simulink model "SICARO"  (R2022b)
settings: Solver=ode23t  StartTime=0.0  StopTime=20  MaxStep=1e-3  RelTol=1e-3  AbsTol=1e-3
values from neighbouring files (symbols this model uses):
  air_rho = 1.225    [sicaro_inherited_params(stall).mat]
  battery_capacity = 22.8    [sicaro_inherited_params(stall).mat]
  CDO = 10.25    [sicaro_inherited_params(stall).mat]
  drag_linear = 0.002    [sicaro_inherited_params(stall).mat]
  drag_quad = 0.005    [sicaro_inherited_params(stall).mat]
  filtD_motor = 100    [sicaro_inherited_params(stall).mat]
  filtSpd_motor = 0.001    [sicaro_inherited_params(stall).mat]
  flap_radius = 0.05312    [sicaro_inherited_params(stall).mat]
  flap_surface_area = 0.025    [sicaro_inherited_params(stall).mat]
  kd_motor = 0    [sicaro_inherited_params(stall).mat]
  ki_motor = 0.00045    [sicaro_inherited_params(stall).mat]
  klinear = 0.03    [sicaro_inherited_params(stall).mat]
  kquad = 0.025    [sicaro_inherited_params(stall).mat]
  limit_motor = 0.25    [sicaro_inherited_params(stall).mat]
  monoco_mass = 160    [sicaro_inherited_params(stall).mat]
  monoco_prop =     [sicaro_inherited_params(stall).mat]
  monoco_radius = 0.61    [sicaro_inherited_params(stall).mat]
  monoco_wing =     [sicaro_inherited_params(stall).mat]
  monoco_wing_area = 0.239    [sicaro_inherited_params(stall).mat]
  waypoints = [-2 -2 0.14 -2 -2 6 0 0 6 2 0 6 ... (15 elements, 3x5)]    [sicaro_inherited_params(stall).mat]
undefined symbols (not defined in the file or in its folder): X, Y, Z
libraries: sm_lib x96, nesl_utility x38, slpidlib x20, fl_lib x12, sdl_lib x3, simulink x2, simulink_extras x1, batteryecm_lib x1, ee_lib x1
(part 7 of 7)

== matlab function SICARO/Collective Control/PD Alt Controller (Monoco positve direction clockwise)/Motor speed 2 thrust plot ==
  data: u input; y output
function y = fcn(u)
coder.extrinsic('fit');
input = u;

%disp (size(u));

%%%%% generate motor plot %%%%%%%%%%
% conversion2rads = 0.10471975513824;
% convert2Newton = 9.81/1000; 
% speed = conversion2rads.*[-31578 -31211 -30294 -29297 -28264 -27239 -26403 -25568 -24568 -23218 -21868 -20546 -19344 -18122 -16851 -15490 -13823 -11985 -8414 0 8414 11985 13823 15490 16851 18122 19334 20546 21868 23218 24568 25568 26403 27239 28264 29297 30294 31211 31578];
% speed = transpose(speed);
% thrust = convert2Newton.*[-485,-475,-450,-425,-400,-375,-350,-325,-300,-275,-250,-225,-200,-175,-150,-125,-100,-75,-50,0,50,75,100,125,150,175,200,225,250,275,300,325,350,375,400,425,450,475,485];
% thrust = transpose(thrust);
% f = fit(speed,thrust,'poly3'); % speed thrust function
% disp (f);
% disp (f(-10));
% plot(f,speed,thrust);
% xlabel('RPS')
% ylabel('Force')
% title('Motor plot force vs speed')

% rps = (100/2290).*[2290 2175.5 2061 1946.5 1832 1717.5 1603 1488.5 1374 1259.5 1145 1030.5 916];
% rps = transpose(rps);
% rot_freq = 0.1591549.*[30.2 28.82 27.5 26.21 24.95 23.71 22.5 21.3 20.13 18.97 17.82 16.67 15.5];
% rot_freq = transpose(rot_freq);
% g = fit(rps,rot_freq,'poly2');  % high thrust = high rotational freq = high lift
% disp(g);
% plot(g,rps,rot_freq);
% xlabel('thrust(%)')
% ylabel('rot_freq(hz)')
% title('thrust vs rot_freq')


x = input; 
func = 7.884e-11*x^3 - 7.663e-12*x^2 + 0.0006131*x + 8.695e-05; % motor speed(rps) vs thrust(N) ~ approximation, this value is the approx motor thrust obtained from motor rps 
y = func;


%y= 0;
% disp("func is");
% disp(y);
% disp("input is");
% disp(input);

== matlab function SICARO/Monowing/Speed Brake mode/Speed Brake Mode Activation ==
  data: rps input; y output; monoco_radius parameter; pitch input; air_rho parameter; monoco_wing_area parameter; Time input; Mode input
function y = fcn(rps, monoco_radius, pitch, air_rho, monoco_wing_area, Time, Mode)
linear_vel_sq = zeros(1,1);
linear_vel_sq = (rps * monoco_radius)^2;
drag_angle = 120;
drag_coeff = 0.1;



if Mode == 0
    if (pitch > drag_angle) && (Time < 8.0) 
        y = 0.5 * drag_coeff * air_rho * monoco_wing_area * linear_vel_sq * monoco_radius;
    else
        y = 0.0;
    end
else
    y = 0.0;
end

== matlab function SICARO/Monowing/Collective Control/Collective (Anhedral) ==
  data: Torque_negative input; Toggle input; output output
function output  = fcn(Torque_negative, Toggle)

if Toggle == 2.0
    output = Torque_negative * 1.0; % change this 
else
    output = 0.0;
end
%y = Torque_negative;

== matlab function SICARO/Monowing/Drag State/Drag filter ==
  data: drag input; Time input; drag_upper output; drag_lower output; Mode input
function [drag_upper, drag_lower] = fcn(drag, Time, Mode)
if Mode == 0
    if Time > 8.0 && Time < 12.0
        drag_upper = drag;
        drag_lower = 0.0;
    elseif Time > 12.0
        drag_lower = -1 * drag;
        drag_upper = 0.0;
    else
        drag_upper = drag;
        drag_lower = 0.0;
    end

elseif Mode == 1
    drag_upper = drag;
    drag_lower = 0.0;

else
    drag_upper = 0.0;
    drag_lower = -1 * drag;

end

== matlab function SICARO/Hover ==
  data: Y output; toggle_y output; X output; toggle_x output; Time input
function [Y, toggle_y, X, toggle_x] = fcn(Time)

sol_X = zeros(1,1);
sol_Toggle_Y = zeros(1,1);
sol_Toggle_X = zeros(1,1);
sol_Y = zeros(1,1);
Velocity = 0.2;

if Time > 10 && Time < 50
%     if Time > 10 && Time < 15
%         sol_X = 0;
%         sol_Toggle_Y = 1;
%         sol_Toggle_X = 1;
%         sol_Y = -1;
%     
%     elseif Time > 15 && Time < 20
%         sol_X = 0;
%         sol_Toggle_Y = 1;
%         sol_Toggle_X = 1;
%         sol_Y = 0;
%     
%     elseif Time > 20 && Time < 25
%         sol_X = 0;
%         sol_Toggle_Y = 1;
%         sol_Toggle_X = 1;
%         sol_Y = 1;
% 
%     elseif Time > 25 && Time < 30
%         sol_X = 0;
%         sol_Toggle_Y = 1;
%         sol_Toggle_X = 1;
%         sol_Y = 0;
%     end
% 
% else
    sol_X = 0;
    sol_Y = 0;
    sol_Toggle_Y = 1;
    sol_Toggle_X = 1;
end

Y = sol_Y;
X = sol_X;
toggle_y = sol_Toggle_Y;
toggle_x = sol_Toggle_X;

== matlab function SICARO/Monowing/Monowing_Assem/Old SICARO Controller For Translation/Collective & Cyclic Command Distribution (Disk Pitch) abt Yw ==
  data: u input; flap_dihedral_pitch_cmd output; gain_x input; heading input; Toggle input; Motor_Pulse output
function [flap_dihedral_pitch_cmd,Motor_Pulse] = fcn(u, gain_x, heading, Toggle)

if Toggle == 1 % Front Motor

    azimuth = u;
    %heading = deg2rad(heading);
    if ((abs(azimuth) - deg2rad(heading)) > pi/4) && ((abs(azimuth) - deg2rad(heading)) < 3*pi/4)
        tilt_xw = sin(azimuth - deg2rad(heading)); % tilt about yw heading in x direction 
        pitch = zeros(1,1);
        pitch = tilt_xw * gain_x; % only for cyclic y
        Motor_Pulse =  (pitch/abs(pitch)) * 1;

        if abs(pitch) > 0.60
            pitch = (pitch/abs(pitch)) * 0.60;
        end

        flap_dihedral_pitch_cmd = pitch;

    else
        
        Motor_Pulse =  0;
        flap_dihedral_pitch_cmd = 0.0;

    end

elseif Toggle == 2 % Back Motor

    azimuth = u;
    if (abs(azimuth) > pi/4) && (abs(azimuth) < 3*pi/4)
        tilt_xw = sin(azimuth + heading); % tilt around xw heading in y direction 
        pitch = zeros(1,1);
        pitch = tilt_xw * gain_x; % only for cyclic y
        Motor_Pulse =  (pitch/abs(pitch)) * 1;

        if abs(pitch) > 0.75
            pitch = (pitch/abs(pitch)) * 0.75;
        end

        flap_dihedral_pitch_cmd = pitch;

    else
        
        Motor_Pulse =  0;
        flap_dihedral_pitch_cmd = 0.0;

    end

else
    
    Motor_Pulse =  0;
    flap_dihedral_pitch_cmd = 0.0;

end





% kp = 1.3;
% desired_roll = 10;
% if (Annular_roll/abs(Annular_roll)) > 0.0
%     error_gain = kp*(Annular_roll - desired_roll);
% 
% elseif (Annular_roll/abs(Annular_roll)) < 0.0
%     error_gain = kp*(Annular_roll - (-1*desired_roll));
% 
% else
%     error_gain = 0.0;
% 
% end

% roll = gain * desired_flap * 2; % only for cyclic (original) 
% roll = desired_flap; % collective
% flap_cmd = roll - error_gain;

== matlab function SICARO/Monowing/Monowing_Assem/Old SICARO Controller For Translation/Cyclic Command Distribution ==
  data: pitch_gain_dihedral_front input; roll_gain_dihedral_front input; pitch_gain_dihedral_back input; roll_gain_dihedral_back input; Transition_Mode output; gain_x output; gain_y output; Dihedral_Mode output; Mode_Selection input
function [Transition_Mode, gain_x, gain_y, Dihedral_Mode] = fcn(pitch_gain_dihedral_front, roll_gain_dihedral_front, pitch_gain_dihedral_back, roll_gain_dihedral_back, Mode_Selection)

if Mode_Selection == 1
    Transition_Mode = 0;
    Dihedral_Mode = 1;
    gain_x = pitch_gain_dihedral_front;
    gain_y = roll_gain_dihedral_front;
else 
    Transition_Mode = 0;
    Dihedral_Mode = 2;
    gain_x = pitch_gain_dihedral_back;
    gain_y = roll_gain_dihedral_back;
end



% if Mode_Selection == 0
%     Transition_Mode = 1;
%     Dihedral_Mode = 0;
%     Anhedral_Mode = 0;
%     gain_x = 0;
%     gain_y = 0;
% elseif Mode_Selection == 1
%     Transition_Mode = 0;
%     Dihedral_Mode = 1;
%     Anhedral_Mode = 0;
%     gain_x = pitch_gain_dihedral;
%     gain_y = roll_gain_dihedral;
% elseif Mode_Selection == 2
%     Transition_Mode = 0;
%     Dihedral_Mode = 0;
%     Anhedral_Mode = 1;
%     gain_x = pitch_gain_anhedral;
%     gain_y = roll_gain_anhedral;
% else 
%     Transition_Mode = 0;
%     Dihedral_Mode = 0;
%     Anhedral_Mode = 0;
%     gain_x = 0;
%     gain_y = 0;
% end

== matlab function SICARO/Monowing/Collective Control/Collective Mode Switcher ==
  data: dihedral output; Time input; anhedral output; Mode input
function [dihedral,anhedral] = fcn(Time,Mode)
if Mode == 1
      dihedral = 1.0;
      anhedral = 0.0;
    
elseif Mode == 2
    dihedral = 1.0;
    anhedral = 0.0;
else
    dihedral = 0.0;
    anhedral = 0.0;
end


% if Mode == 0
%     
%     if Time > 8.0 && Time < 12.0
%         dihedral = 0.0; % upside cut torque
%         anhedral = 0.0;
%     elseif Time > 10
%         dihedral = 0.0;
%         anhedral = 1.0;
%     else
%         dihedral = 1.0;
%         anhedral = 0.0;
%     end
% 
% elseif Mode == 1
% 
%     dihedral = 1.0;
%     anhedral = 0.0;
% 
% elseif Mode == 2
% 
%     dihedral = 0.0;
%     anhedral = 1.0;
% 
% else
% 
%     dihedral = 0.0;
%     anhedral = 0.0;
% 
% end

== matlab function SICARO/Monowing/Horizontal Forces/Horizontal Motion X ==
  data: roll_in_deg input; force output; Lift input; flap_angle_data input; vx input; vy input; vz input; klinear parameter; kquad parameter; azimuth input; flap_angle input; desired_heading input; active_state output
function [force,active_state]  = fcn(roll_in_deg, Lift, flap_angle_data, vx, vy, vz, klinear, kquad, azimuth, flap_angle, desired_heading)
fx = zeros(1,1);
x = zeros(1,1);
v_l1 = zeros(1,1);
v_l2 = zeros(1,1);
roll_angle = abs(roll_in_deg);
%disp(Lift);
dihedral_offset = 2.0;
v_l1 = abs(vx) + abs(vy) + abs(vz);
v_l2 = sqrt(vx^2 + vy^2 + vz^2);

negative_x = 0;
positive_x = 1;
neutral_x = 2;
desired_heading = deg2rad(desired_heading);

if (azimuth - desired_heading) > 0 && flap_angle > 0 
    current_state = negative_x;
    active_state = 1;

elseif (azimuth - desired_heading) < 0 && flap_angle < 0
    current_state = negative_x;
    active_state = 2;
    
elseif (azimuth - desired_heading) > pi && flap_angle < 0
    current_state = negative_x;
    active_state = 3;

elseif (azimuth - desired_heading) > 0 && flap_angle < 0
    current_state = positive_x;
    active_state = 4;

elseif (azimuth - desired_heading) < 0 && flap_angle > 0
    current_state = positive_x;
    active_state = 5;

elseif (azimuth - desired_heading) > pi && flap_angle > 0
    current_state = positive_x;
    active_state = 6;

else
    current_state = neutral_x;
    active_state = 0;
end

%disp (current_state);
% disp (azimuth);
% disp (flap_angle);

% current_state = negative_y;

switch(current_state)

    case negative_x
        if roll_in_deg > 0 && roll_in_deg > dihedral_offset 
        %     if roll_in_deg > 0
            fx = Lift*sind(roll_in_deg-dihedral_offset);
            x = (-1*fx) + (kquad*v_l1*abs(vy) + klinear*abs(vy));
        elseif roll_in_deg < 0
            fx = Lift*sind(roll_angle);
            x = (-1*fx) + (kquad*v_l1*abs(vy) + klinear*abs(vy));
            %y = y  (kquad*v_l1*abs(vy) + klinear*abs(vy));
        else
            x = 0.0;
        end

    case positive_x
        if roll_in_deg > 0 && roll_in_deg > dihedral_offset 
        %     if roll_in_deg > 0
            fx = Lift*sind(roll_in_deg-dihedral_offset);
            x = fx - (kquad*v_l1*abs(vy) + klinear*abs(vy));
        elseif roll_in_deg < 0
            fx = Lift*sind(roll_angle);
            x = fx - (kquad*v_l1*abs(vy) + klinear*abs(vy));
            %y = y  (kquad*v_l1*abs(vy) + klinear*abs(vy));
        else
            x = 0.0;
        end

    case neutral_x 
            x = 0.0;

end

force = x;
% Acceleration_in_x_axis = x/monoco_mass;
% flap_angle_recording = flap_angle_data;

== matlab function SICARO/Monowing/Monowing_Assem/Old SICARO Controller For Translation/Collective & Cyclic Command Distribution (Disk Roll) abt Xw ==
  data: u input; flap_dihedral_roll_cmd output; gain_y input; heading input; Toggle input; Motor_Pulse output
function [flap_dihedral_roll_cmd,Motor_Pulse] = fcn(u, gain_y, heading, Toggle)

if Toggle == 1 % Front Motor

    azimuth = u;
    if (abs(azimuth) > 3*pi/4) || (abs(azimuth) < pi/4)
        tilt_yw = cos(azimuth + heading); % tilt around xw heading in y direction 
        roll = zeros(1,1);
        roll = tilt_yw * gain_y; % only for cyclic y
        Motor_Pulse =  (roll/abs(roll)) * 1;

        if abs(roll) > 0.6
            roll = (roll/abs(roll)) * 0.6;
        end

        flap_dihedral_roll_cmd = roll;

    else
        
        Motor_Pulse =  0;
        flap_dihedral_roll_cmd = 0.0;

    end

elseif Toggle == 2 % Back Motor

    azimuth = u;
    if (abs(azimuth) > 3*pi/4) || (abs(azimuth) < pi/4)
        tilt_yw = cos(azimuth + heading); % tilt around xw heading in y direction 
        roll = zeros(1,1);
        roll = tilt_yw * gain_y; % only for cyclic y
        Motor_Pulse =  (roll/abs(roll)) * 1;

        if abs(roll) > 0.6
            roll = (roll/abs(roll)) * 0.6;
        end

        flap_dihedral_roll_cmd = roll;

    else
        
        Motor_Pulse =  0;
        flap_dihedral_roll_cmd = 0.0;

    end

else
    
    Motor_Pulse =  0;
    flap_dihedral_roll_cmd = 0.0;

end







% kp = 1.3;
% desired_roll = 10;
% if (Annular_roll/abs(Annular_roll)) > 0.0
%     error_gain = kp*(Annular_roll - desired_roll);
% 
% elseif (Annular_roll/abs(Annular_roll)) < 0.0
%     error_gain = kp*(Annular_roll - (-1*desired_roll));
% 
% else
%     error_gain = 0.0;
% 
% end

% roll = gain * desired_flap * 2; % only for cyclic (original) 
% roll = desired_flap; % collective
% flap_cmd = roll - error_gain;

== matlab function SICARO/Cyclic Roll Control/PD Roll Controller (Monoco negative direction counter clockwise) Front Motor/Gain Switching ==
  data: aggro input; y output; Toggle input; annular_roll input; gentle input
function y = fcn(aggro, Toggle, annular_roll, gentle)

if Toggle > 0
    if abs(annular_roll) > 5.0
        y = aggro;
    else
        y = gentle;
    end
else
    y = 0;
end

% y = gentle;

== matlab function SICARO/Diamond ==
  data: Y output; toggle_y output; X output; toggle_x output; Time input; Z output
function [Y, toggle_y, X, toggle_x, Z] = fcn(Time)

sol_X = zeros(1,1);
sol_Toggle_Y = zeros(1,1);
sol_Toggle_X = zeros(1,1);
sol_Y = zeros(1,1);
Velocity = 0.35;

z = 2.3; 
if Time > 10 && Time < 37
    if Time > 10 && Time < 16
        sol_X = -2;
        sol_Toggle_Y = 1;
        sol_Toggle_X = 1;
        sol_Y = 2;
        z = 2.3; 
    
    elseif Time > 16 && Time < 27
        sol_X = 2;
        sol_Toggle_Y = 1;
        sol_Toggle_X = 1;
        sol_Y = 2;
        z = 2.0; 
    
    elseif Time > 27 && Time < 33
        sol_X = 0;
        sol_Toggle_Y = 1;
        sol_Toggle_X = 1;
        sol_Y = 0;
        z = 2.0; 
    end

else
    sol_X = 0;
    sol_Y = 0;
    sol_Toggle_Y = 0;
    sol_Toggle_X = 0;
end

Y = sol_Y;
X = sol_X;
Z = z;
toggle_y = sol_Toggle_Y;
toggle_x = sol_Toggle_X;

== matlab function SICARO/Motor speed 2 motor induced torque plot (Back Motor) ==
  data: u input; y output; Mode input
function y = fcn(u, Mode)
coder.extrinsic('fit');
input = u;

%disp (size(u));

%%%%% generate motor torque %%%%%%%%%%
% speed = [-8414 -11985 -13823 -15490 -16851 -18122 -19334 -20546 -21868 -23218 -24568 -25568 -26403 -27239 -28264 -29297 -30294 -31211 -31578 0 8414 11985 13823 15490 16851 18122 19334 20546 21868 23218 24568 25568 26403 27239 28264 29297 30294 31211 31578];
% %speed = transpose(speed);
% power = [-14.88 -21.18 -31 -41.67 -53.85 -66.98 -80.75 -94.53 -110.53 -127.1 -143.66 -161.84 -180.78 -199.72 -213.16 -226.38 -243.4 -268.51 -279.30 0 14.88 21.18 31 41.67 53.85 66.98 80.75 94.53 110.53 127.1 143.66 161.84 180.78 199.72 213.16 226.38 243.4 268.51 279.30];
% %power = transpose(power);
% torque = mrdivide(power,speed);
% %torque = transpose(torque);
% disp(torque);

% f = fit(speed,torque,'poly3'); % speed torque function
% disp (f);
% disp (f(-10));
% plot(f,speed,torque);
% xlabel('RPM')
% ylabel('Torque')
% title('Motor plot torque vs speed')


% conversion2rpm = 0.10471975513824;
% x = abs(input)/conversion2rpm; 
if Mode == 2
    y = 0.0031 * -1;  % dun change!
else
    y = 0.0031 * 0;
end
 
    
% y = 0.0066 * 0;

%y= 0;
% disp("func is");
% disp(y);
% disp("input is");
% disp(input);

== matlab function SICARO/Square Trajectory ==
  data: Y output; toggle_y output; X output; toggle_x output; Time input
function [Y, toggle_y, X, toggle_x] = fcn(Time)

sol_X = zeros(1,1);
sol_Toggle_Y = zeros(1,1);
sol_Toggle_X = zeros(1,1);
sol_Y = zeros(1,1);
Velocity = 0.2;

if Time > 6 && Time < 120
    if Time > 6 && Time < 16
        sol_X = 2;
        sol_Toggle_Y = 1;
        sol_Toggle_X = 1;
        sol_Y = 0;
    
    elseif Time > 16 && Time < 26
        sol_X = 2;
        sol_Toggle_Y = 1;
        sol_Toggle_X = 1;
        sol_Y = 4;
    
    elseif Time > 26 && Time < 36
        sol_X = -2;
        sol_Toggle_Y = 1;
        sol_Toggle_X = 1;
        sol_Y = 4;
    
    elseif Time > 32 && Time < 42
        sol_X = -2;
        sol_Toggle_Y = 1;
        sol_Toggle_X = 1;
        sol_Y = 0;
    
    elseif Time > 42 && Time < 50
        sol_X = 0;
        sol_Toggle_Y = 1;
        sol_Toggle_X = 1;
        sol_Y = 0;
    end

else
    sol_X = 0;
    sol_Y = 0;
    sol_Toggle_Y = 0;
    sol_Toggle_X = 0;
end

Y = sol_Y;
X = sol_X;
toggle_y = sol_Toggle_Y;
toggle_x = sol_Toggle_X;

== matlab function SICARO/Monowing/flap_moment  ==
  data: flap_angle input; y output; rps input; monoco_radius parameter; air_rho parameter; flap_surface_area parameter; flap_radius parameter
function y = fcn(flap_angle, rps, monoco_radius, air_rho, flap_surface_area, flap_radius)
linear_vel_sq = zeros(1,1);
linear_vel_sq = (rps * monoco_radius)^2;
y = flap_radius * 0.5 * 0.005 * flap_angle * air_rho * flap_surface_area * linear_vel_sq;

== matlab function SICARO/Motor speed 2 motor induced torque plot (Front Motor) ==
  data: u input; y output; Mode input
function y = fcn(u, Mode)
coder.extrinsic('fit');
input = u;

%disp (size(u));

%%%%% generate motor plot %%%%%%%%%%
% speed = [-8414 -11985 -13823 -15490 -16851 -18122 -19334 -20546 -21868 -23218 -24568 -25568 -26403 -27239 -28264 -29297 -30294 -31211 -31578 0 8414 11985 13823 15490 16851 18122 19334 20546 21868 23218 24568 25568 26403 27239 28264 29297 30294 31211 31578];
% %speed = transpose(speed);
% power = [-14.88 -21.18 -31 -41.67 -53.85 -66.98 -80.75 -94.53 -110.53 -127.1 -143.66 -161.84 -180.78 -199.72 -213.16 -226.38 -243.4 -268.51 -279.30 0 14.88 21.18 31 41.67 53.85 66.98 80.75 94.53 110.53 127.1 143.66 161.84 180.78 199.72 213.16 226.38 243.4 268.51 279.30];
% %power = transpose(power);
% torque = mrdivide(power,speed);
% %torque = transpose(torque);
% disp(torque);

% f = fit(speed,torque,'poly3'); % speed torque function
% disp (f);
% disp (f(-10));
% plot(f,speed,torque);
% xlabel('RPM')
% ylabel('Torque')
% title('Motor plot torque vs speed')


% conversion2rpm = 0.10471975513824;
% x = abs(input)/conversion2rpm; 
if Mode == 1
    y = 0.0031 * 1; % dun change!
else
    %y = 0.0066 * 0;
    y = 0.0031 * 0; 
end    
% y = 0.0066 * 0;

%y= 0;
% disp("func is");
% disp(y);
% disp("input is");
% disp(input);

== matlab function SICARO/Cyclic Roll Control/PD Pitch Controller (Monoco negative direction counter clockwise) Front Motor/Gain Switching2 ==
  data: aggro input; y output; Toggle input; annular_roll input; gentle input
function y = fcn(aggro, Toggle, annular_roll, gentle)

if Toggle > 0
    if abs(annular_roll) > 5.0
        y = aggro;
    else
        y = gentle;
    end
else
    y = 0;
end


% y = gentle;

== matlab function SICARO/Collective Control/PD Alt Controller (Monoco negative direction counter clockwise)/Motor Pulsing Filter ==
  data: u input; y output; toggle input
function y = fcn(u, toggle)

motor_pulse = zeros(1,1);

if toggle == 1
    motor_pulse = -1 * abs(u);
elseif toggle == -1
    motor_pulse = abs(u);
else
    motor_pulse = 0;
end

if abs(motor_pulse) > 300
    motor_pulse = motor_pulse/abs(motor_pulse) * 300;

end

y = motor_pulse;

== matlab function SICARO/Y Test ==
  data: Y output; toggle_y output; X output; toggle_x output; Time input
function [Y, toggle_y, X, toggle_x] = fcn(Time)

sol_X = zeros(1,1);
sol_Toggle_Y = zeros(1,1);
sol_Toggle_X = zeros(1,1);
sol_Y = zeros(1,1);
Velocity = 0.2;

if Time > 10 && Time < 40
   if Time > 10 && Time < 18
        sol_X = 0;
        sol_Toggle_Y = 1;
        sol_Toggle_X = 0;
        sol_Y = -2;
    
    elseif Time > 18 && Time < 30
        sol_X = 0;
        sol_Toggle_Y = 1;
        sol_Toggle_X = 0;
        sol_Y = 2;
    
    elseif Time > 30 && Time < 40
        sol_X = 0;
        sol_Toggle_Y = 1;
        sol_Toggle_X = 0;
        sol_Y = 0;
    end

else
    sol_X = 0;
    sol_Y = 0;
    sol_Toggle_Y = 1;
    sol_Toggle_X = 1;
end

Y = sol_Y;
X = sol_X;
toggle_y = sol_Toggle_Y;
toggle_x = sol_Toggle_X;

== matlab function SICARO/X Test ==
  data: Y output; toggle_y output; X output; toggle_x output; Time input
function [Y, toggle_y, X, toggle_x] = fcn(Time)

sol_X = zeros(1,1);
sol_Toggle_Y = zeros(1,1);
sol_Toggle_X = zeros(1,1);
sol_Y = zeros(1,1);
Velocity = 0.2;

if Time > 10 && Time < 40
    if Time > 10 && Time < 18
        sol_X = -2;
        sol_Toggle_Y = 0;
        sol_Toggle_X = 1;
        sol_Y = 0;
    
    elseif Time > 18 && Time < 30
        sol_X = 2;
        sol_Toggle_Y = 0;
        sol_Toggle_X = 1;
        sol_Y = 0;
    
    elseif Time > 30 && Time < 40
        sol_X = 0;
        sol_Toggle_Y = 0;
        sol_Toggle_X = 1;
        sol_Y = 0;
    end

else
    sol_X = 0;
    sol_Y = 0;
    sol_Toggle_Y = 0;
    sol_Toggle_X = 0;
end

Y = sol_Y;
X = sol_X;
toggle_y = sol_Toggle_Y;
toggle_x = sol_Toggle_X;

== matlab function SICARO/Cyclic Roll Control/PD Roll Controller (Monoco negative direction counter clockwise) Back Motor/Gain Switching ==
  data: aggro input; y output; Toggle input; annular_roll input; gentle input
function y = fcn(aggro, Toggle, annular_roll, gentle)

if Toggle > 0
    if abs(annular_roll) > 5
        y = aggro;
    else
        y = gentle;
    end
else
    y = 0;
end

% y = gentle;

== matlab function SICARO/Collective Control/PD Alt Controller (Monoco negative direction counter clockwise)/Motor speed 2 thrust plot ==
  data: u input; y output
function y = fcn(u)
coder.extrinsic('fit');
input = u;

%disp (size(u));

%%%%% generate motor plot %%%%%%%%%%
% conversion2rads = 0.10471975513824;
% convert2Newton = 9.81/1000; 
% speed = conversion2rads.*[-31578 -31211 -30294 -29297 -28264 -27239 -26403 -25568 -24568 -23218 -21868 -20546 -19344 -18122 -16851 -15490 -13823 -11985 -8414 0 8414 11985 13823 15490 16851 18122 19334 20546 21868 23218 24568 25568 26403 27239 28264 29297 30294 31211 31578];
% speed = transpose(speed);
% thrust = convert2Newton.*[-485,-475,-450,-425,-400,-375,-350,-325,-300,-275,-250,-225,-200,-175,-150,-125,-100,-75,-50,0,50,75,100,125,150,175,200,225,250,275,300,325,350,375,400,425,450,475,485];
% thrust = transpose(thrust);
% f = fit(speed,thrust,'poly3'); % speed thrust function
% disp (f);
% disp (f(-10));
% plot(f,speed,thrust);
% xlabel('RPS')
% ylabel('Force')
% title('Motor plot force vs speed')

% rps = (100/2290).*[2290 2175.5 2061 1946.5 1832 1717.5 1603 1488.5 1374 1259.5 1145 1030.5 916];
% rps = transpose(rps);
% rot_freq = 0.1591549.*[30.2 28.82 27.5 26.21 24.95 23.71 22.5 21.3 20.13 18.97 17.82 16.67 15.5];
% rot_freq = transpose(rot_freq);
% g = fit(rps,rot_freq,'poly2');  % high thrust = high rotational freq = high lift
% disp(g);
% plot(g,rps,rot_freq);
% xlabel('thrust(%)')
% ylabel('rot_freq(hz)')
% title('thrust vs rot_freq')


x = input; 
% prev % func = 7.884e-11*x^3 - 7.663e-12*x^2 + 0.0006131*x + 8.695e-05; % motor speed(rps) vs thrust(N) ~ approximation, this value is the approx motor thrust obtained from motor rps
func = 4.975e-11*x^3 + 3.747e-23*x^2 + 0.0003889*x - 3.142e-16;
y = func;


%y= 0;
% disp("func is");
% disp(y);
% disp("input is");
% disp(input);

== matlab function SICARO/Cyclic Roll Control/PD Pitch Controller (Monoco negative direction counter clockwise)2/Gain Switching2 ==
  data: aggro input; y output; Toggle input; annular_roll input; gentle input
function y = fcn(aggro, Toggle, annular_roll, gentle)

if Toggle > 0
    if abs(annular_roll) < 2.75
        y = aggro;
    else
        y = gentle;
    end
else
    y = 0;
end

== matlab function SICARO/Cyclic Roll Control/PD Pitch Controller (Monoco negative direction counter clockwise) Back Motor/Gain Switching2 ==
  data: aggro input; y output; Toggle input; annular_roll input; gentle input
function y = fcn(aggro, Toggle, annular_roll, gentle)

if Toggle > 0
    if abs(annular_roll) > 5.0
        y = aggro;
    else
        y = gentle;
    end
else
    y = 0;
end

% y = gentle;

== matlab function SICARO/Square Trajectory1 ==
  data: Y output; toggle_y output; X output; toggle_x output; Time input
function [Y, toggle_y, X, toggle_x] = fcn(Time)

sol_X = zeros(1,1);
sol_Toggle_Y = zeros(1,1);
sol_Toggle_X = zeros(1,1);
sol_Y = zeros(1,1);
Velocity = 0.2;

if Time > 6 && Time < 120
    if Time > 6 && Time < 16
        sol_X = 2;
        sol_Toggle_Y = 1;
        sol_Toggle_X = 1;
        sol_Y = 0;
    
    elseif Time > 16 && Time < 26
        sol_X = 2;
        sol_Toggle_Y = 1;
        sol_Toggle_X = 1;
        sol_Y = 4;
    
    elseif Time > 26 && Time < 36
        sol_X = -2;
        sol_Toggle_Y = 1;
        sol_Toggle_X = 1;
        sol_Y = 4;
    
    elseif Time > 32 && Time < 42
        sol_X = -2;
        sol_Toggle_Y = 1;
        sol_Toggle_X = 1;
        sol_Y = 0;
    
    elseif Time > 42 && Time < 50
        sol_X = 0;
        sol_Toggle_Y = 1;
        sol_Toggle_X = 1;
        sol_Y = 0;
    end

else
    sol_X = 0;
    sol_Y = 0;
    sol_Toggle_Y = 0;
    sol_Toggle_X = 0;
end

Y = sol_Y;
X = sol_X;
toggle_y = sol_Toggle_Y;
toggle_x = sol_Toggle_X;

== matlab function SICARO/Polar Test Front Motor ==
  data: mag_setpt output; Time input; desired_heading output; toggle output
function [mag_setpt, desired_heading, toggle] = fcn(Time)

mag = zeros(1,1);
heading = zeros(1,1);
cyclic_toggle = zeros(1,1);
% this is an exceptional example  

if Time > 10 && Time < 40
    cyclic_toggle = 1;
    if Time > 10 && Time < 18
        X_setpoint = -2;
        Y_setpoint = -2;
        mag = sqrt(X_setpoint^2 + Y_setpoint^2);
        
        % originally, supposed to be y as adjacent (due to matlab atan2
        % function structure), but this arrangement of
        % y being the opposite instead due to the swapping solves this issue 
        % atan2(x,y) swap to atan2(y,x)
        heading = atan2(Y_setpoint,X_setpoint);   

    elseif Time > 18 && Time < 26
        X_setpoint = 0-(-2);
        Y_setpoint = 0-(-2);
        mag = sqrt(X_setpoint^2 + Y_setpoint^2);

        % originally, supposed to be y as adjacent (due to matlab atan2
        % function structure), but this arrangement of
        % y being the opposite instead due to the swapping solves this issue 
        % atan2(x,y) swap to atan2(y,x)
        heading = atan2(Y_setpoint,X_setpoint);   
    
%     elseif Time > 26 && Time < 34
%         X_setpoint = 2;
%         Y_setpoint = -2;
%         mag = sqrt(X_setpoint^2 + Y_setpoint^2);
% 
%         % originally, supposed to be y as adjacent (due to matlab atan2
%         % function structure), but this arrangement of
%         % y being the opposite instead due to the swapping solves this issue 
%         % atan2(x,y) swap to atan2(y,x)
%         heading = atan2(Y_setpoint,X_setpoint);
% 
%      elseif Time > 34 && Time < 42
%         X_setpoint = -2;
%         Y_setpoint = 2;
%         mag = sqrt(X_setpoint^2 + Y_setpoint^2);
% 
%         % originally, supposed to be y as adjacent (due to matlab atan2
%         % function structure), but this arrangement of
%         % y being the opposite instead due to the swapping solves this issue 
%         % atan2(x,y) swap to atan2(y,x)
%         heading = atan2(Y_setpoint,X_setpoint);

    end
else
    cyclic_toggle = 0;
    mag = 0;
    heading = 0;
end
toggle = cyclic_toggle;
mag_setpt = mag;
desired_heading = heading;

== matlab function SICARO/Cyclic Roll Control/PD Control (Disk-Pitch Body-Roll Front Motor)/Gain Switching ==
  data: aggro input; y output; annular_roll input; gentle input; Toggle input
function y = fcn(aggro, annular_roll, gentle,Toggle)

if Toggle > 0
    if abs(annular_roll) > 5
        y = aggro;
    else
        y = gentle;
    end
else
    y = 0;
end

% y = gentle;

== matlab function SICARO/Cyclic Roll Control/Cartesian to polar transformation ==
  data: polar_feedback output; Y_fb input; X_fb input
function polar_feedback  = fcn(Y_fb,X_fb)

polarfb = zeros(1,1);
polarfb = sqrt(Y_fb^2 + X_fb^2);
polar_feedback = polarfb;

== matlab function SICARO/Monowing/Monowing_Assem/Disk-Pitch Body-Roll Command Distribution ==
  data: Disk_Pitch_Body_Roll_Front input; Disk_Pitch_Body_Roll_Back input; Transition_Mode output; gain output; Mode_Select output; Mode_Selection input
function [Transition_Mode, gain, Mode_Select] = fcn(Disk_Pitch_Body_Roll_Front,Disk_Pitch_Body_Roll_Back,Mode_Selection)

if Mode_Selection == 1
    Transition_Mode = 0;
    Mode_Select = 1;
    gain = Disk_Pitch_Body_Roll_Front;
else 
    Transition_Mode = 0;
    Mode_Select = 2;
    gain = Disk_Pitch_Body_Roll_Back;
end



% if Mode_Selection == 0
%     Transition_Mode = 1;
%     Dihedral_Mode = 0;
%     Anhedral_Mode = 0;
%     gain_x = 0;
%     gain_y = 0;
% elseif Mode_Selection == 1
%     Transition_Mode = 0;
%     Dihedral_Mode = 1;
%     Anhedral_Mode = 0;
%     gain_x = pitch_gain_dihedral;
%     gain_y = roll_gain_dihedral;
% elseif Mode_Selection == 2
%     Transition_Mode = 0;
%     Dihedral_Mode = 0;
%     Anhedral_Mode = 1;
%     gain_x = pitch_gain_anhedral;
%     gain_y = roll_gain_anhedral;
% else 
%     Transition_Mode = 0;
%     Dihedral_Mode = 0;
%     Anhedral_Mode = 0;
%     gain_x = 0;
%     gain_y = 0;
% end

== matlab function SICARO/Monowing/Quat2Eul Function ==
  data: u input; Euler_Angles_Collectively output size=[1 4] [-1000..1000]; bod_pitch_deg_abt_Xb output size=[1,1]; bod_roll_deg_abt_Yb output; body_yaw_rad_z output; Pos output size=[1 5]; Time input; pos_x input; pos_y input; pos_z input; rps input
function [Euler_Angles_Collectively, bod_pitch_deg_abt_Xb, bod_roll_deg_abt_Yb, body_yaw_rad_z, Pos] = fcn(u, Time, pos_x, pos_y, pos_z, rps)
coder.extrinsic('quat2eul');
anx = zeros(1,3);
dax = zeros(1,3);
body_pitch_deg = zeros(1,1);
body_roll_deg = zeros(1,1);
yaw_rad = zeros(1,1);
default_heading = zeros(1,1); % zero heading is at body yb facing world yw 
quat = flip(transpose(u));
% disp (quat);

eul = quat2eul(quat); % ZYX 
% Z = zeros(1,1);

% Body frame dynamics
Z = eul(1,1);
Y = eul(1,2);
X = eul(1,3);
body_pitch_deg = rad2deg(X);
body_roll_deg = rad2deg(Y);
% yaw_deg = rad2deg(Z);
yaw_rad = Z;

anx = rad2deg([X Y Z]);
Pos = [Time pos_x pos_y pos_z rps];
% disp (size(deg));
% disp (size(Z));
Euler_Angles_Collectively = [Time, anx];

% World frame dynamics
% annular_pitch_deg_abt_yw = -1*body_pitch_deg; % anti clockwise is negative but i negate it so its easier to read; annular y axis in world frame
% annular_roll_deg_abt_xw = 1*body_roll_deg; % clockwise is positive; annular x axis in world frame

% Body frame dynamics in euler
bod_pitch_deg_abt_Xb = -1*body_pitch_deg;
bod_roll_deg_abt_Yb = 1*body_roll_deg;
body_yaw_rad_z = yaw_rad;

% Disk frame dynamics in euler (ZYX)
dax = deg2rad([0 bod_roll_deg_abt_Yb 0]);

== matlab function SICARO/Monowing/Monowing_Assem/Collective & Cyclic Command Distribution (Disk-Pitch Body-Roll) abt Yw ==
  data: azi input; flap_dihedral_pitch_cmd output; gain_disk_pitch input; heading input; Toggle input; Motor_Pulse output
function [flap_dihedral_pitch_cmd,Motor_Pulse] = fcn(azi, gain_disk_pitch, heading, Toggle)

if Toggle == 1 % Front Motor

    azimuth = azi;
    %heading = deg2rad(heading);
    if ((abs(azimuth) - deg2rad(heading)) > pi/4) && ((abs(azimuth) - deg2rad(heading)) < 3*pi/4)
        tilt_xw = sin(azimuth - deg2rad(heading)); % tilt about yw heading in x direction 
        pitch = zeros(1,1);
        pitch = tilt_xw * gain_disk_pitch; % only for cyclic y
        Motor_Pulse =  (pitch/abs(pitch)) * 1;

        if abs(pitch) > 0.60
            pitch = (pitch/abs(pitch)) * 0.60;
        end

        flap_dihedral_pitch_cmd = pitch;

    else
        
        Motor_Pulse =  0;
        flap_dihedral_pitch_cmd = 0.0;

    end

elseif Toggle == 2 % Back Motor

    azimuth = azi;
    if (abs(azimuth) > pi/4) && (abs(azimuth) < 3*pi/4)
        tilt_xw = sin(azimuth + heading); % tilt around xw heading in y direction 
        pitch = zeros(1,1);
        pitch = tilt_xw * gain_disk_pitch; % only for cyclic y
        Motor_Pulse =  (pitch/abs(pitch)) * 1;

        if abs(pitch) > 0.75
            pitch = (pitch/abs(pitch)) * 0.75;
        end

        flap_dihedral_pitch_cmd = pitch;

    else
        
        Motor_Pulse =  0;
        flap_dihedral_pitch_cmd = 0.0;

    end

else
    
    Motor_Pulse =  0;
    flap_dihedral_pitch_cmd = 0.0;

end





% kp = 1.3;
% desired_roll = 10;
% if (Annular_roll/abs(Annular_roll)) > 0.0
%     error_gain = kp*(Annular_roll - desired_roll);
% 
% elseif (Annular_roll/abs(Annular_roll)) < 0.0
%     error_gain = kp*(Annular_roll - (-1*desired_roll));
% 
% else
%     error_gain = 0.0;
% 
% end

% roll = gain * desired_flap * 2; % only for cyclic (original) 
% roll = desired_flap; % collective
% flap_cmd = roll - error_gain;

== matlab function SICARO/Monowing/Monowing_Assem/Old SICARO Controller For Translation/Collective & Cyclic Command Distribution (Transition) ==
  data: stalling_flap input; flap_transition_cmd output; Time input; Toggle input
function flap_transition_cmd = fcn(stalling_flap,Time, Toggle)
if Toggle == 1
    
    roll = zeros(1,1);
    roll = stalling_flap; % collective
    
    if Time > 8.0
        flap_transition_cmd = 0.0;
    else 
        flap_transition_cmd = roll;
    end

else

    flap_transition_cmd = 0.0;

end

== matlab function SICARO/Monowing/Drag moment/Drag Moment (X & Y) ==
  data: y input; drag_moment_abt_y output; drag_linear parameter; drag_quad parameter; x input; drag_moment_abt_x output; azimuth input
function [drag_moment_abt_y,drag_moment_abt_x] = fcn(y, drag_linear, drag_quad, x, azimuth)
drag_moment_y  = zeros(1,1);
drag_moment_x  = zeros(1,1);
gain = cos(azimuth);
drag_moment_y = (drag_linear * y) + (drag_quad * y^2); 
drag_moment_x = (drag_linear * x) + (drag_quad * x^2); 

drag_moment_abt_y = -1 * drag_moment_y;
drag_moment_abt_x = -1 * drag_moment_x;

== matlab function SICARO/Monowing/Horizontal Forces/Horizontal Motion Y ==
  data: roll_in_deg input; force output; Lift input; flap_angle_data input; flap_angle_recording output; vx input; vy input; vz input; klinear parameter; kquad parameter; desired_heading input; azimuth input; flap_angle input; active_state output
function [force, flap_angle_recording,active_state] = fcn(roll_in_deg, Lift, flap_angle_data, vx, vy, vz, klinear, kquad, desired_heading, azimuth, flap_angle)
fy = zeros(1,1);
y = zeros(1,1);
v_l1 = zeros(1,1);
v_l2 = zeros(1,1);
roll_angle = abs(roll_in_deg);
%disp(Lift);
dihedral_offset = 2.0;
v_l1 = abs(vx) + abs(vy) + abs(vz);
v_l2 = sqrt(vx^2 + vy^2 + vz^2);

negative_y = 0;
positive_y = 1;
neutral_y = 2;
desired_heading = deg2rad(desired_heading);

if (abs(azimuth) - desired_heading) < pi/2 && flap_angle > 0 
    current_state = negative_y; % positive y with z axis facing in
    active_state = 1;
    
elseif (abs(azimuth) - desired_heading) > pi/2 && flap_angle < 0
    current_state = negative_y; % positive y with z axis facing in
    active_state = 2;

elseif (abs(azimuth) - desired_heading) > pi/2 && flap_angle > 0
    current_state = positive_y; % negative y with z axis facing in
    active_state = 3;

elseif (abs(azimuth) - desired_heading) < pi/2 && flap_angle < 0
    current_state = positive_y; % negative y with z axis facing in
    active_state = 4;

else
    current_state = neutral_y;
    active_state = 0;
end

% disp (current_state);
% disp (azimuth);
% disp (flap_angle);

% current_state = negative_y;

switch(current_state)
    % positive y with z axis facing in  
    case negative_y
        if roll_in_deg > 0 && roll_in_deg > dihedral_offset 
        %     if roll_in_deg > 0
            fy = Lift*sind(roll_in_deg-dihedral_offset);
            y = (-1*fy) + (kquad*v_l1*abs(vy) + klinear*abs(vy));
        elseif roll_in_deg < 0
            fy = Lift*sind(roll_angle);
            y = (-1*fy) + (kquad*v_l1*abs(vy) + klinear*abs(vy));
            %y = y  (kquad*v_l1*abs(vy) + klinear*abs(vy));
        else
            y = 0.0;
        end
    % negative y with z axis facing in
    case positive_y
        if roll_in_deg > 0 && roll_in_deg > dihedral_offset 
        %     if roll_in_deg > 0
            fy = Lift*sind(roll_in_deg-dihedral_offset);
            y = fy - (kquad*v_l1*abs(vy) + klinear*abs(vy));
        elseif roll_in_deg < 0
            fy = Lift*sind(roll_angle);
            y = fy - (kquad*v_l1*abs(vy) + klinear*abs(vy));
            %y = y  (kquad*v_l1*abs(vy) + klinear*abs(vy));
        else
            y = 0.0;
        end

    case neutral_y 
            y = 0.0;

end

force = y;
% Acceleration_in_y_axis = y/monoco_mass;
flap_angle_recording = flap_angle_data;

== matlab function SICARO/Monowing/Collective Control/Collective (Dihedral) ==
  data: Torque_negative input; output output; Toggle input
function output  = fcn(Torque_negative,Toggle)

if Toggle == 1 
    output = Torque_negative;
else
    output = 0;
end
